simulink model "zynqRadioHWSWLTEDetectorAD9361AD9364SL"  (R2016a)
settings: Solver=FixedStepDiscrete  SolverMode=SingleTasking  StartTime=0.0  StopTime=inf  RelTol=1e-3
InitFcn:
  | % Load LTE detector initialization parameters
  | simParams = hdlcoder_lteofdm_modDetectref_init;
  | simParams = hdlcoder_lteofdm_modDetecthdl_init(simParams);
  | 
  | % Modify PSS detection threshold gain for modified
  | % front-end filter
  | simParams.thresholdGain = 16;
  | 
  | % Load LTE TX waveforms
  | load('zynqRadioLTETransmitData');
libraries: simulink x26, hdlsllib x18, dspsigops x3, dspxfrm3 x1, dspmlti4 x1, dspmathops x1, dspsrcs4 x1
(part 1 of 2)
CloseFcn:
  | clear simParams;
settings Model: DataTypeOverride=Off  SimulationMode=accelerator  Creator=The MathWorks, Inc.  LastModifiedBy=The MathWorks, Inc.
settings DataIOCC: LimitDataPoints=on  SaveFormat=Array  SaveOutput=off  VisualizeSimOutput=off  SaveTime=off
settings OptimizationCC: BlockReduction=off  BooleanDataType=off  ConditionallyExecuteInputs=off  DefaultParameterBehavior=Inlined  EfficientMapNaN2IntZero=off
settings DebuggingCC: AlgebraicLoopMsg=error  SaveWithParameterizedLinksMsg=none  UnderspecifiedInitializationDetection=Classic  MergeDetectMultiDrivingBlocksExec=none  SignalResolutionControl=TryResolveAllWithWarning  SingleTaskRateTransMsg=error  ParameterPrecisionLossMsg=none  AllowSymbolicDim=off  StrictBusMsg=ErrorOnBusTreatedAsVector
settings HardwareCC: ProdBitPerPointer=32  ProdLargestAtomicFloat=None  ProdIntDivRoundTo=Undefined  ProdEndianess=Unspecified  ProdWordSize=32  ProdHWDeviceType=ASIC/FPGA->ASIC/FPGA  TargetBitPerPointer=64  TargetLongLongMode=on  TargetIntDivRoundTo=Zero  TargetEndianess=LittleEndian  TargetWordSize=64  TargetHWDeviceType=MATLAB Host  ProdEqTarget=off
settings ModelReferenceCC: PropagateSignalLabelsOutOfModel=off
settings CodeAppCC: MaxIdLength=128
settings GRTTargetCC: GeneratePreprocessorConditionals=Use local settings  CombineOutputUpdateFcns=off  GRTInterface=on
settings ConfigComp: CovSFcnEnable=off

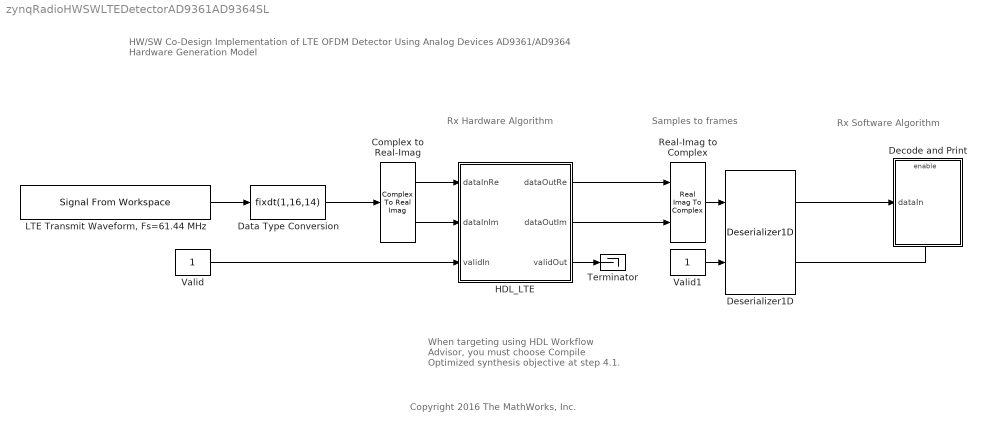
== system zynqRadioHWSWLTEDetectorAD9361AD9364SL ==
  note: When targeting using HDL Workflow Advisor, you must choose Compile Optimized synthesis objective at step 4.1.
  note: HW/SW Co-Design Implementation of LTE OFDM Detector Using Analog Devices AD9361/AD9364
      | Hardware Generation Model
  note: Copyright 2016 The MathWorks, Inc.
  note: Rx Software Algorithm
  note: Rx Hardware Algorithm
  note: Samples to frames
  Complex to Real-Imag : ComplexToRealImag
  Data Type Conversion : DataTypeConversion  OutDataTypeStr=fixdt(1,16,14)
  Decode and Print : Subsystem
  Deserializer1D : hdlsllib/HDL Operations/Deserializer1D  Ratio=5000  IdleCycles=0  InitialCondition=0  startIn=off  validIn=on  validOut=on  inputDataDimensions=1  inputSampleTime=-1  inputSignalType=auto
  HDL_LTE : Subsystem  TreatAsAtomicUnit=on
  "LTE Transmit Waveform, Fs=61.44 MHz" : dspsrcs4/Signal From Workspace  X=zynqRadioLTETransmitData_CellID_16  Ts=1/61.44e6  nsamps=1  OutputAfterFinalValue=Cyclic repetition  ignoreOrWarnInputAndFrameLengths=off  OutputFrames=off
  Real-Imag to Complex : RealImagToComplex
  Terminator : Terminator
  Valid : Constant  VectorParams1D=off  OutDataTypeStr=boolean  SampleTime=1/61.44e6
  Valid1 : Constant  VectorParams1D=off  OutDataTypeStr=boolean  SampleTime=1/61.44e6
  wires:
  "LTE Transmit Waveform, Fs=61.44 MHz"/1 -> Data Type Conversion/1
  Complex to Real-Imag/1 -> HDL_LTE/1(dataInRe)
  Complex to Real-Imag/2 -> HDL_LTE/2(dataInIm)
  HDL_LTE/1(dataOutRe) -> Real-Imag to Complex/1
  HDL_LTE/2(dataOutIm) -> Real-Imag to Complex/2
  Real-Imag to Complex/1 -> Deserializer1D/1
  Deserializer1D/1 -> Decode and Print/1(dataIn)
  Deserializer1D/2 -> Decode and Print/Enable
  Data Type Conversion/1 -> Complex to Real-Imag/1
  Valid/1 -> HDL_LTE/3(validIn)
  Valid1/1 -> Deserializer1D/2
  HDL_LTE/3(validOut) -> Terminator/1

== system zynqRadioHWSWLTEDetectorAD9361AD9364SL/Decode and Print ==
  dataIn : Inport
  Enable : EnablePort
  PrintCellID : MATLAB Function  TreatAsAtomicUnit=on
  wires:
  dataIn/1 -> PrintCellID/1(u)

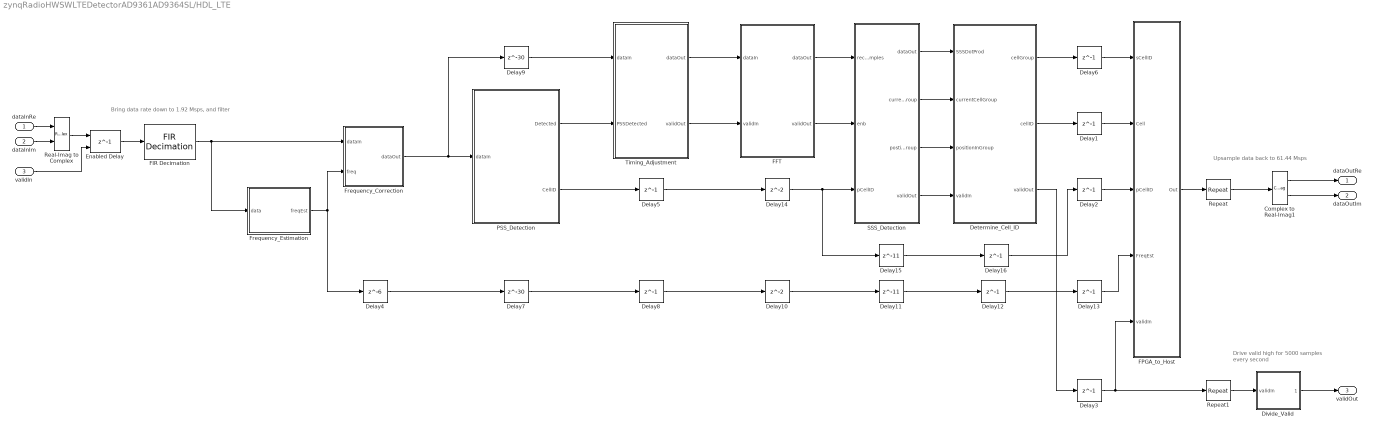
== system zynqRadioHWSWLTEDetectorAD9361AD9364SL/HDL_LTE ==
  note: Drive valid high for 5000 samples
      | every second
  note: Upsample data back to 61.44 Msps
  note: Bring data rate down to 1.92 Msps, and filter
  dataInRe : Inport
  dataInIm : Inport  Port=2
  validIn : Inport  Port=3
  Complex to Real-Imag1 : ComplexToRealImag
  Delay{1..3,5..6,8,12..13,16} (9 alike) : Delay  DelayLength=1  InitialCondition=0  UseCircularBuffer=on
  Delay10 : Delay  InitialCondition=0  UseCircularBuffer=on
  Delay11 : Delay  DelayLength=11  InitialCondition=0  UseCircularBuffer=on
  Delay14 : Delay  InitialCondition=0  UseCircularBuffer=on
  Delay15 : Delay  DelayLength=11  InitialCondition=0  UseCircularBuffer=on
  Delay4 : Delay  DelayLength=6  InitialCondition=0  UseCircularBuffer=on
  Delay7 : Delay  DelayLength=30  InitialCondition=0  InputProcessing=Columns as channels (frame based)
  Delay9 : Delay  DelayLength=30  InitialCondition=0  InputProcessing=Columns as channels (frame based)
  Determine_Cell_ID : Subsystem
  Divide_Valid : Subsystem  mask{cnt=61.44e6, frameSize=5000}
      mask prompts: cnt "Count Value"; frameSize "Frame Size"
  Enabled Delay : Delay  DelayLength=1  ShowEnablePort=on
      settings: InputPortMap=u0,e6
  FFT : Subsystem
  FIR Decimation : dspmlti4/FIR Decimation  FilterSource=Dialog parameters  h="[-0.00658036135584628\t0.0196845728924509\t0.0188740770712237\t0.0238501032851229\t0.0307518159057901\t0.0383679693229666\t0.0461438771533022\t0.0536253945544419\t0.0604305519429808\t0.0661752266061415\t0.0705384318505213\t0.0732639414365212\t0.0741823592553149\t0.0732639414365212\t0.0705384318505213\t0.0661752266061415\t0.0604305519429808\t0.0536253945544419\t0.0461438771533022\t0.0383679693229666\t0.0307518159057901\t0.0238501032851229\t0.0188740770712237\t0.0196845728924509\t-0.00658036135584628]"  D=32  filtStruct=Direct form transposed  FilterObject=FDECIM  framing=Enforce single-rate processing  inputOffset=0  outputBufInitCond=0  roundingMode=Floor  overflowMode=off  firstCoeffDataTypeStr=Inherit: Same word length as input  firstCoeffMin=[]  firstCoeffMax=[]  firstCoeffLastDataTypeStr=Inherit: Same word length as input  outputMin=[]  outputMax=[]
  FPGA_to_Host : Subsystem
  Frequency_Correction : Subsystem
  Frequency_Estimation : Subsystem
  PSS_Detection : Subsystem
  Real-Imag to Complex : RealImagToComplex
  Repeat : dspsigops/Repeat  N=32  RateOptions=Allow multirate processing  ic=0  mode=Unused parameter value
  Repeat1 : dspsigops/Repeat  N=32  RateOptions=Allow multirate processing  ic=0  mode=Unused parameter value
  SSS_Detection : Subsystem
  Timing_Adjustment : Subsystem
  dataOutRe : Outport
  dataOutIm : Outport  Port=2
  validOut : Outport  Port=3  PortDimensions=1
  wires:
  Delay6/1 -> FPGA_to_Host/1(sCellID)
  FPGA_to_Host/1(Out) -> Repeat/1
  Delay1/1 -> FPGA_to_Host/2(Cell)
  Timing_Adjustment/2(validOut) -> FFT/2(validIn)
  FFT/2(validOut) -> SSS_Detection/2(enb)
  Delay9/1 -> Timing_Adjustment/1(dataIn)
  FFT/1(dataOut) -> SSS_Detection/1(receiveSamples)
  Timing_Adjustment/1(dataOut) -> FFT/1(dataIn)
  SSS_Detection/1(dataOut) -> Determine_Cell_ID/1(SSSDotProd)
  SSS_Detection/2(currentCellGroup) -> Determine_Cell_ID/2(currentCellGroup)
  SSS_Detection/3(postionInGroup) -> Determine_Cell_ID/3(positionInGroup)
  PSS_Detection/2(CellID) -> Delay5/1
  PSS_Detection/1(Detected) -> Timing_Adjustment/2(PSSDetected)
  Frequency_Correction/1(dataOut) -> Delay9/1, PSS_Detection/1(dataIn)
  Frequency_Estimation/1(freqEst) -> Frequency_Correction/2(freq), Delay4/1
  Determine_Cell_ID/1(cellGroup) -> Delay6/1
  Determine_Cell_ID/2(cellID) -> Delay1/1
  Delay2/1 -> FPGA_to_Host/3(pCellID)
  Enabled Delay/1 -> FIR Decimation/1
  Real-Imag to Complex/1 -> Enabled Delay/1
  dataInRe/1 -> Real-Imag to Complex/1
  dataInIm/1 -> Real-Imag to Complex/2
  validIn/1 -> Enabled Delay/2
  Repeat/1 -> Complex to Real-Imag1/1
  Complex to Real-Imag1/1 -> dataOutRe/1
  Complex to Real-Imag1/2 -> dataOutIm/1
  SSS_Detection/4(validOut) -> Determine_Cell_ID/4(validIn)
  Determine_Cell_ID/3(validOut) -> Delay3/1
  Delay3/1 -> Repeat1/1, FPGA_to_Host/5(validIn)
  Delay4/1 -> Delay7/1
  Delay7/1 -> Delay8/1
  Delay8/1 -> Delay10/1
  Delay10/1 -> Delay11/1
  Delay11/1 -> Delay12/1
  Delay12/1 -> Delay13/1
  Delay14/1 -> SSS_Detection/3(pCellID), Delay15/1
  Delay15/1 -> Delay16/1
  Delay16/1 -> Delay2/1
  Delay5/1 -> Delay14/1
  Delay13/1 -> FPGA_to_Host/4(FreqEst)
  Divide_Valid/1(validOut) -> validOut/1
  Repeat1/1 -> Divide_Valid/1(validIn)
  FIR Decimation/1 -> Frequency_Estimation/1(data), Frequency_Correction/1(dataIn)

== system zynqRadioHWSWLTEDetectorAD9361AD9364SL/HDL_LTE/Determine_Cell_ID ==
  note: N_ID(2)
  note: Calculate detected Cell ID
      | (CellID = 3*N_ID(1) + N_ID(2))
  note: N_ID(1)
  note: If incoming SSS correlation output is greater than that stored in register,
      | store new maximum value, and cell group number, in registers
  note: Store maximum value in register
  note: Store corresponding cell group in register
  SSSDotProd : Inport
  currentCellGroup : Inport  Port=2
  positionInGroup : Inport  Port=3
  validIn : Inport  Port=4
  Add2 : Sum  OutDataTypeStr=Inherit: Same as first input
  Delay3 : Delay  DelayLength=1  InitialCondition=0  UseCircularBuffer=on
  Gain1 : Gain  Gain=3  OutDataTypeStr=fixdt(0,9,0)
  Relational Operator4 : RelationalOperator  Operator=>  OutDataTypeStr=boolean
  Unit Delay Enabled1 : simulink/Additional Math & Discrete/Additional Discrete/Unit Delay Enabled  vinit=0  tsamp=-1
  Unit Delay Enabled3 : simulink/Additional Math & Discrete/Additional Discrete/Unit Delay Enabled  vinit=0  tsamp=-1
  cellGroup : Outport
  cellID : Outport  Port=2
  validOut : Outport  Port=3
  wires:
  Add2/1 -> cellID/1
  SSSDotProd/1 -> Unit Delay Enabled3/1, Relational Operator4/1
  positionInGroup/1 -> Add2/2
  Unit Delay Enabled1/1 -> Gain1/1, cellGroup/1
  currentCellGroup/1 -> Unit Delay Enabled1/1
  Relational Operator4/1 -> Unit Delay Enabled3/2, Unit Delay Enabled1/2
  Gain1/1 -> Add2/1
  Unit Delay Enabled3/1 -> Relational Operator4/2
  validIn/1 -> Delay3/1
  Delay3/1 -> validOut/1

== system zynqRadioHWSWLTEDetectorAD9361AD9364SL/HDL_LTE/Divide_Valid ==
  validIn : Inport
  Compare To Constant : simulink/Logic and Bit Operations/Compare To Constant  relop=>  const=cnt-frameSize-1  OutDataTypeStr=boolean
  HDL Counter : hdlsllib/HDL Operations/HDL Counter  CountType=Count limited  CountInit=0  CountStep=1  CountMax=cnt-1  CountFromType=Initial value  CountFrom=0  CountResetPort=off  CountLoadPort=off  CountEnbPort=on  CountDirPort=off  CountDataType=Unsigned  CountWordLen=ceil(log2(cnt))  CountFracLen=0  CountSampTime=1
  validOut : Outport
  wires:
  Compare To Constant/1 -> validOut/1
  HDL Counter/1 -> Compare To Constant/1
  validIn/1 -> HDL Counter/1

== system zynqRadioHWSWLTEDetectorAD9361AD9364SL/HDL_LTE/FFT ==
  note: Set input of FFT to input wordlength + FFT growth to allow
      | the output of the FFT to scale. Maximum bit growth is equal
      | to log2(nFFT).
  dataIn : Inport
  validIn : Inport  Port=2
  Data Type Conversion : DataTypeConversion  OutDataTypeStr=fixdt(1,18,10)  RndMeth=Round
  Delay{1..2,4..5} (4 alike) : Delay  DelayLength=1  InitialCondition=0  InputProcessing=Columns as channels (frame based)
  FFT HDL Optimized : dspxfrm3/FFT HDL Optimized  Architecture=Streaming Radix 2 (this choice will be removed -see release notes).  ComplexMultiplication=Use 3 multipliers and 5 adders  BitReversedOutput=off  Normalize=off  FFTLength=128  RoundingMethod=Floor  ResetInputPort=off  StartOutputPort=off  EndOutputPort=off  SimulateUsing=Code generation
  Signal Specification : SignalSpecification  Dimensions=1
  Signal Specification1 : SignalSpecification  Dimensions=1
  dataOut : Outport
  validOut : Outport  Port=2
  wires:
  Signal Specification1/1 -> FFT HDL Optimized/2
  Signal Specification/1 -> FFT HDL Optimized/1
  FFT HDL Optimized/2 -> Delay5/1
  FFT HDL Optimized/1 -> Delay4/1
  Delay4/1 -> Data Type Conversion/1
  Delay2/1 -> Signal Specification1/1
  dataIn/1 -> Delay1/1
  validIn/1 -> Delay2/1
  Delay1/1 -> Signal Specification/1
  Data Type Conversion/1 -> dataOut/1
  Delay5/1 -> validOut/1

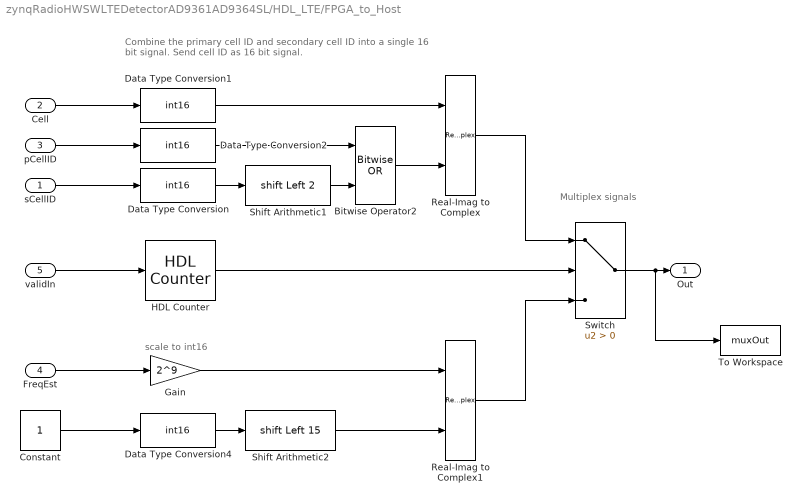
== system zynqRadioHWSWLTEDetectorAD9361AD9364SL/HDL_LTE/FPGA_to_Host ==
  note: Multiplex signals
  note: scale to int16
  note: Combine the primary cell ID and secondary cell ID into a single 16 bit signal. Send cell ID as 16 bit signal.
  sCellID : Inport
  Cell : Inport  Port=2
  pCellID : Inport  Port=3
  FreqEst : Inport  Port=4
  validIn : Inport  Port=5
  Bitwise Operator2 : simulink/Logic and Bit Operations/Bitwise Operator  logicop=OR  UseBitMask=off  NumInputPorts=2  BitMask=bin2dec('11011001')  BitMaskRealWorld=Stored Integer
  Constant : Constant  VectorParams1D=off  OutDataTypeStr=boolean  SampleTime=-1
  Data Type Conversion{,1..2,4} (4 alike) : DataTypeConversion  OutDataTypeStr=int16
  Gain : Gain  Gain=2^9  OutDataTypeStr=int16
  HDL Counter : hdlsllib/HDL Operations/HDL Counter  CountType=Count limited  CountInit=0  CountStep=1  CountMax=1  CountFromType=Initial value  CountFrom=0  CountResetPort=off  CountLoadPort=off  CountEnbPort=on  CountDirPort=off  CountDataType=Unsigned  CountWordLen=1  CountFracLen=0  CountSampTime=1
  Real-Imag to Complex : RealImagToComplex
  Real-Imag to Complex1 : RealImagToComplex
  Shift Arithmetic1 : ArithShift  BitShiftNumber=2  BitShiftDirection=Left
  Shift Arithmetic2 : ArithShift  BitShiftNumber=15  BitShiftDirection=Left
  Switch : Switch  Criteria=u2 > Threshold
  To Workspace : ToWorkspace  VariableName=muxOut  SampleTime=-1
      settings: Save2DSignal=2-D array (concatenate along first dimension)
  Out : Outport
  wires:
  Data Type Conversion2/1 -> Bitwise Operator2/1
  Data Type Conversion/1 -> Shift Arithmetic1/1
  Bitwise Operator2/1 -> Real-Imag to Complex/2
  Shift Arithmetic1/1 -> Bitwise Operator2/2
  Data Type Conversion1/1 -> Real-Imag to Complex/1
  Cell/1 -> Data Type Conversion1/1
  sCellID/1 -> Data Type Conversion/1
  pCellID/1 -> Data Type Conversion2/1
  Switch/1 -> To Workspace/1, Out/1
  FreqEst/1 -> Gain/1
  validIn/1 -> HDL Counter/1
  HDL Counter/1 -> Switch/2
  Real-Imag to Complex/1 -> Switch/1
  Gain/1 -> Real-Imag to Complex1/1
  Shift Arithmetic2/1 -> Real-Imag to Complex1/2
  Constant/1 -> Data Type Conversion4/1
  Data Type Conversion4/1 -> Shift Arithmetic2/1
  Real-Imag to Complex1/1 -> Switch/3

== system zynqRadioHWSWLTEDetectorAD9361AD9364SL/HDL_LTE/Frequency_Correction ==
  note: This subsystem corrects the frequency offset using an Numerically Controller Oscillator (NCO) and a conjugate multiplication.
  dataIn : Inport
  freq : Inport  Port=2
  Data Type Conversion : DataTypeConversion  OutDataTypeStr=fixdt(1,16,15)  RndMeth=Nearest
  Delay{1..6} (6 alike) : Delay  DelayLength=1  InitialCondition=0  UseCircularBuffer=on
  Gain : Gain  Gain=2^9  OutDataTypeStr=int16
  NCO HDL Optimized : dspsigops/NCO HDL Optimized  PhaseIncrementSource=Input port  PhaseIncrement=100  PhaseOffsetSource=Property  PhaseOffset=0  DitherSource=Property  NumDitherBits=4  PhaseQuantization=on  NumQuantizerAccumulatorBits=12  LUTCompress=on  ResetAction=off  ValidInputPort=off  Waveform=Complex exponential  PhasePort=off  AccumulatorWL=16  OutputDataType=Binary point scaling  OutputWL=16  OutputFL=14  SimulateUsing=Code generation
  Product1 : Product
  Signal Spec : SignalSpecification  Dimensions=1
  Unit Delay Enabled : simulink/Additional Math & Discrete/Additional Discrete/Unit Delay Enabled  vinit=0.0  tsamp=-1
  complexConjugate : Math  Operator=conj  SaturateOnIntegerOverflow=on
  dataOut : Outport
  wires:
  complexConjugate/1 -> Delay3/1
  NCO HDL Optimized/2 -> Unit Delay Enabled/2
  dataIn/1 -> Delay2/1
  Product1/1 -> Delay4/1
  NCO HDL Optimized/1 -> Unit Delay Enabled/1
  Unit Delay Enabled/1 -> complexConjugate/1
  Data Type Conversion/1 -> Delay1/1
  Delay2/1 -> Product1/1
  Delay1/1 -> dataOut/1
  Delay4/1 -> Data Type Conversion/1
  Delay3/1 -> Product1/2
  Gain/1 -> Delay5/1
  freq/1 -> Delay6/1
  Delay6/1 -> Gain/1
  Signal Spec/1 -> NCO HDL Optimized/1
  Delay5/1 -> Signal Spec/1

== system zynqRadioHWSWLTEDetectorAD9361AD9364SL/HDL_LTE/Frequency_Estimation ==
  data : Inport
  Angle_Filter : Subsystem
  Angle_at_Maximum : Subsystem
  Cyclic_Prefix_Correlator : Subsystem
  Rect_to_Polar : Subsystem
  freqEst : Outport
  wires:
  data/1 -> Cyclic_Prefix_Correlator/1(dataIn)
  Rect_to_Polar/3(validOut) -> Angle_at_Maximum/3(validIn)
  Angle_at_Maximum/1(angleOut) -> Angle_Filter/1(angleIn)
  Rect_to_Polar/2(angleOut) -> Angle_at_Maximum/2(angleIn)
  Rect_to_Polar/1(magOut) -> Angle_at_Maximum/1(magIn)
  Cyclic_Prefix_Correlator/1(corrOut) -> Rect_to_Polar/1(dataIn)
  Angle_Filter/1(angleOut) -> freqEst/1
  Angle_at_Maximum/2(validOut) -> Angle_Filter/2(en)

== system zynqRadioHWSWLTEDetectorAD9361AD9364SL/HDL_LTE/PSS_Detection ==
  dataIn : Inport
  Cross_Correlation : Subsystem
  Determine_Primary_Cell_ID : Subsystem
  Peak_Detection : Subsystem
  Detected : Outport
  CellID : Outport  Port=2
  wires:
  Determine_Primary_Cell_ID/1(Cell_ID) -> CellID/1
  Determine_Primary_Cell_ID/2(PSSDetected) -> Detected/1
  Cross_Correlation/1(PSS0) -> Peak_Detection/1(PSS0)
  Cross_Correlation/2(PSS1) -> Peak_Detection/2(PSS1)
  Cross_Correlation/3(PSS2) -> Peak_Detection/3(PSS2)
  Cross_Correlation/4(Threshold) -> Peak_Detection/4(thresholdIn)
  Peak_Detection/2(PSS0Strength) -> Determine_Primary_Cell_ID/2(PSS0Strength)
  Peak_Detection/4(PSS1Strength) -> Determine_Primary_Cell_ID/4(PSS1Strength)
  Peak_Detection/5(PSS2Detected) -> Determine_Primary_Cell_ID/5(PSS2Detected)
  Peak_Detection/6(PSS2Strength) -> Determine_Primary_Cell_ID/6(PSS2Strength)
  Peak_Detection/1(PSS0Detected) -> Determine_Primary_Cell_ID/1(PSS0Detected)
  Peak_Detection/3(PSS1Detected) -> Determine_Primary_Cell_ID/3(PSS1Detected)
  dataIn/1 -> Cross_Correlation/1(dataIn)

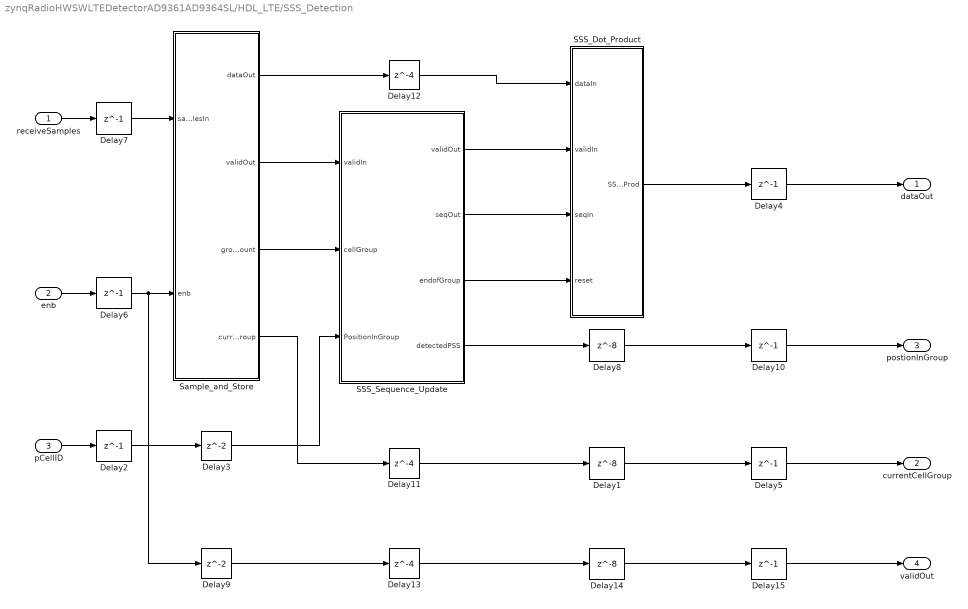
== system zynqRadioHWSWLTEDetectorAD9361AD9364SL/HDL_LTE/SSS_Detection ==
  receiveSamples : Inport
  enb : Inport  Port=2
  pCellID : Inport  Port=3
  Delay1 : Delay  DelayLength=8  InitialCondition=0  UseCircularBuffer=on
  Delay{2,4..7,10,15} (7 alike) : Delay  DelayLength=1  InitialCondition=0  UseCircularBuffer=on
  Delay11 : Delay  DelayLength=4  InitialCondition=0
  Delay12 : Delay  DelayLength=4  InitialCondition=0
  Delay13 : Delay  DelayLength=4  InitialCondition=0
  Delay14 : Delay  DelayLength=8  InitialCondition=0  UseCircularBuffer=on
  Delay3 : Delay  InitialCondition=0
  Delay8 : Delay  DelayLength=8  InitialCondition=0  UseCircularBuffer=on
  Delay9 : Delay  InitialCondition=0
  SSS_Dot_Product : Subsystem
  SSS_Sequence_Update : Subsystem
  Sample_and_Store : Subsystem
  dataOut : Outport
  currentCellGroup : Outport  Port=2
  postionInGroup : Outport  Port=3
  validOut : Outport  Port=4
  wires:
  SSS_Dot_Product/1(SSSDotProd) -> Delay4/1
  Delay3/1 -> SSS_Sequence_Update/3(PositionInGroup)
  Sample_and_Store/3(groupCount) -> SSS_Sequence_Update/2(cellGroup)
  Delay2/1 -> Delay3/1
  enb/1 -> Delay6/1
  receiveSamples/1 -> Delay7/1
  pCellID/1 -> Delay2/1
  Sample_and_Store/2(validOut) -> SSS_Sequence_Update/1(validIn)
  Delay7/1 -> Sample_and_Store/1(samplesIn)
  Delay6/1 -> Delay9/1, Sample_and_Store/2(enb)
  Sample_and_Store/1(dataOut) -> Delay12/1
  SSS_Sequence_Update/1(validOut) -> SSS_Dot_Product/2(validIn)
  SSS_Sequence_Update/2(seqOut) -> SSS_Dot_Product/3(seqIn)
  SSS_Sequence_Update/3(endofGroup) -> SSS_Dot_Product/4(reset)
  SSS_Sequence_Update/4(detectedPSS) -> Delay8/1
  Delay8/1 -> Delay10/1
  Delay1/1 -> Delay5/1
  Delay10/1 -> postionInGroup/1
  Delay5/1 -> currentCellGroup/1
  Delay4/1 -> dataOut/1
  Sample_and_Store/4(currentCellGroup) -> Delay11/1
  Delay11/1 -> Delay1/1
  Delay12/1 -> SSS_Dot_Product/1(dataIn)
  Delay9/1 -> Delay13/1
  Delay13/1 -> Delay14/1
  Delay14/1 -> Delay15/1
  Delay15/1 -> validOut/1

== system zynqRadioHWSWLTEDetectorAD9361AD9364SL/HDL_LTE/Timing_Adjustment ==
  note: Detect PSS detection strobe, and create
      | valid high signal.
  note: Delay signal so that once the PSS
      | has been detected, the resource block
      | containing the SSS signal (the previous
      | block) is aligned here.
  note: Only output samples once
      | the detected strobe has
      | been received.
  note: PSS detect strobe is high at the end of the PSS
      | sequence, so delay must be for the full 128 samples
      | of the PSS, and the full 128 samples of the SSS, plus
      | a single short CP length of 9 samples for 128-point
      | FFT.
  dataIn : Inport
  PSSDetected : Inport  Port=2
  Constant : Constant  Value=complex(0)  OutDataTypeStr=fixdt(1,16,15)  SampleTime=simParams.TsRx
  Constant1 : Constant  OutDataTypeStr=boolean  SampleTime=simParams.TsRx
  Delay1 : Delay  DelayLength=265  InitialCondition=0  InputProcessing=Columns as channels (frame based)
  Delay{2..5} (4 alike) : Delay  DelayLength=1  InitialCondition=0  UseCircularBuffer=on
  Switch : Switch  Criteria=u2 > Threshold
  Unit Delay Enabled1 : simulink/Additional Math & Discrete/Additional Discrete/Unit Delay Enabled  vinit=0.0  tsamp=-1
  dataOut : Outport
  validOut : Outport  Port=2
  wires:
  Delay5/1 -> validOut/1
  Delay4/1 -> dataOut/1
  Delay3/1 -> Delay1/1
  Delay2/1 -> Unit Delay Enabled1/2
  Constant/1 -> Switch/3
  Delay1/1 -> Switch/1
  dataIn/1 -> Delay3/1
  Switch/1 -> Delay4/1
  PSSDetected/1 -> Delay2/1
  Unit Delay Enabled1/1 -> Switch/2, Delay5/1
  Constant1/1 -> Unit Delay Enabled1/1

== system zynqRadioHWSWLTEDetectorAD9361AD9364SL/HDL_LTE/Frequency_Estimation/Angle_Filter ==
  note: This subsystem implements a 1-pole IIR filter to perform further averaging of the correlation angle results. The filter's gain is normalized to 0dB and an efficient implementation which requires only 1 multiplier is used.
  angleIn : Inport
  en : Inport  Port=2
  Add : Sum  Inputs=|-+
  Add1 : Sum  Inputs=|-+
  Delay1 : Delay  DelayLength=1  InitialCondition=0  UseCircularBuffer=on
  Delay2 : Delay  DelayLength=1  InitialCondition=0  UseCircularBuffer=on
  Delay3 : Delay  DelayLength=1  InitialCondition=0  UseCircularBuffer=on
  Gain : Gain  Gain=2^-2  OutDataTypeStr=Inherit: Same as input
  Unit Delay Enabled : simulink/Additional Math & Discrete/Additional Discrete/Unit Delay Enabled  vinit=0.0  tsamp=-1
  angleOut : Outport
  wires:
  angleIn/1 -> Delay2/1
  Add/1 -> Gain/1
  Gain/1 -> Add1/1
  Unit Delay Enabled/1 -> Add/2, Add1/2, Delay1/1
  Add1/1 -> Unit Delay Enabled/1
  en/1 -> Delay3/1
  Delay1/1 -> angleOut/1
  Delay2/1 -> Add/1
  Delay3/1 -> Unit Delay Enabled/2

== system zynqRadioHWSWLTEDetectorAD9361AD9364SL/HDL_LTE/Frequency_Estimation/Angle_at_Maximum ==
  note: This subsystem records the maximum CP correlation level, and the corresponding phase angle of the result, across windows of time equivalent to 1 slot (960 samples). A counter is used to reset the running max and record the final phase value, which is then passed to the output and qualified by the validOut signal.
  note: Store current mag & angle if mag is greater than previous max mag.
  note: This register stores the current running max magnitude in the current time window
  magIn : Inport
  angleIn : Inport  Port=2
  validIn : Inport  Port=3
  Compare To Constant : simulink/Logic and Bit Operations/Compare To Constant  relop===  const=0  OutDataTypeStr=boolean
  Delay{1..3,5} (4 alike) : Delay  DelayLength=1  InitialCondition=0  UseCircularBuffer=on
  HDL Counter : hdlsllib/HDL Operations/HDL Counter  CountType=Count limited  CountInit=0  CountStep=1  CountMax=959  CountFromType=Initial value  CountFrom=0  CountResetPort=off  CountLoadPort=off  CountEnbPort=on  CountDirPort=off  CountDataType=Unsigned  CountWordLen=10  CountFracLen=0  CountSampTime=1
  Logical Operator : Logic  Operator=OR  IconShape=distinctive  AllPortsSameDT=off  OutDataTypeStr=boolean
  Relational Operator : RelationalOperator  Operator=>  OutDataTypeStr=boolean
  Unit Delay Enabled : simulink/Additional Math & Discrete/Additional Discrete/Unit Delay Enabled  vinit=0.0  tsamp=-1
  Unit Delay Enabled1 : simulink/Additional Math & Discrete/Additional Discrete/Unit Delay Enabled  vinit=0.0  tsamp=-1
  Unit Delay Enabled2 : simulink/Additional Math & Discrete/Additional Discrete/Unit Delay Enabled  vinit=0.0  tsamp=-1
  angleOut : Outport
  validOut : Outport  Port=2
  wires:
  magIn/1 -> Delay5/1
  angleIn/1 -> Delay1/1
  HDL Counter/1 -> Compare To Constant/1
  Compare To Constant/1 -> Unit Delay Enabled2/2, Logical Operator/2, Delay3/1
  Unit Delay Enabled1/1 -> Unit Delay Enabled2/1
  validIn/1 -> Delay2/1
  Delay5/1 -> Relational Operator/1, Unit Delay Enabled/1
  Delay2/1 -> HDL Counter/1
  Unit Delay Enabled2/1 -> angleOut/1
  Delay3/1 -> validOut/1
  Unit Delay Enabled/1 -> Relational Operator/2
  Relational Operator/1 -> Logical Operator/1
  Logical Operator/1 -> Unit Delay Enabled1/2, Unit Delay Enabled/2
  Delay1/1 -> Unit Delay Enabled1/1

== system zynqRadioHWSWLTEDetectorAD9361AD9364SL/HDL_LTE/Frequency_Estimation/Cyclic_Prefix_Correlator ==
  note: Correlate the signal with itself
      | delayed by the FFT length (128 samples).
  note: Integrate across part of the CP length, which is 9 samples. However we use 8 samples here to optimize for HDL implementation.
  note: Finally average across 7 OFDM symbols, i.e. the number in
      | each slot.
  dataIn : Inport
  Delay1 : Delay  DelayLength=1  InitialCondition=0  UseCircularBuffer=on
  Delay2 : Delay  DelayLength=128  InitialCondition=0
  Delay3 : Delay  DelayLength=1  InitialCondition=0  UseCircularBuffer=on
  Delay5 : Delay  DelayLength=1  InitialCondition=0  UseCircularBuffer=on
  Moving_Average : Subsystem
  Product : Product  OutDataTypeStr=fixdt(1,24,23)  RndMeth=Round
  Slot_Average : Subsystem
  complexConj : Math  Operator=conj  SaturateOnIntegerOverflow=on
  corrOut : Outport
  wires:
  Product/1 -> Delay5/1
  Delay3/1 -> Product/2
  Delay2/1 -> complexConj/1
  Slot_Average/1(dataOut) -> corrOut/1
  Moving_Average/1(dataOut) -> Slot_Average/1(dataIn)
  complexConj/1 -> Delay3/1
  Delay5/1 -> Moving_Average/1(dataIn)
  Delay1/1 -> Product/1
  dataIn/1 -> Delay2/1, Delay1/1

== system zynqRadioHWSWLTEDetectorAD9361AD9364SL/HDL_LTE/Frequency_Estimation/Rect_to_Polar ==
  dataIn : Inport
  Complex to Magnitude-Angle HDL Optimized : dspmathops/Complex to Magnitude-Angle HDL Optimized  NumIterationsSource=Auto  NumIterations=16  OutputFormat=Magnitude and angle  AngleFormat=Normalized  ScaleOutput=on  SimulateUsing=Code generation
  Constant : Constant  OutDataTypeStr=boolean  SampleTime=simParams.TsRx
  Delay1 : Delay  InitialCondition=0  UseCircularBuffer=on
  Delay2 : Delay  DelayLength=1  InitialCondition=0  UseCircularBuffer=on
  Delay3 : Delay  DelayLength=1  InitialCondition=0  UseCircularBuffer=on
  Delay4 : Delay  DelayLength=1  InitialCondition=0  UseCircularBuffer=on
  Delay5 : Delay  InitialCondition=0  UseCircularBuffer=on
  Gain : Gain  Gain=0.5  OutDataTypeStr=fixdt(1,27,27)
  Signal Specification1 : SignalSpecification  Dimensions=1
  magOut : Outport
  angleOut : Outport  Port=2
  validOut : Outport  Port=3
  wires:
  Gain/1 -> angleOut/1
  dataIn/1 -> Signal Specification1/1
  Constant/1 -> Delay1/1
  Delay5/1 -> Complex to Magnitude-Angle HDL Optimized/1
  Delay1/1 -> Complex to Magnitude-Angle HDL Optimized/2
  Delay2/1 -> magOut/1
  Delay3/1 -> Gain/1
  Delay4/1 -> validOut/1
  Complex to Magnitude-Angle HDL Optimized/1 -> Delay2/1
  Complex to Magnitude-Angle HDL Optimized/3 -> Delay4/1
  Complex to Magnitude-Angle HDL Optimized/2 -> Delay3/1
  Signal Specification1/1 -> Delay5/1

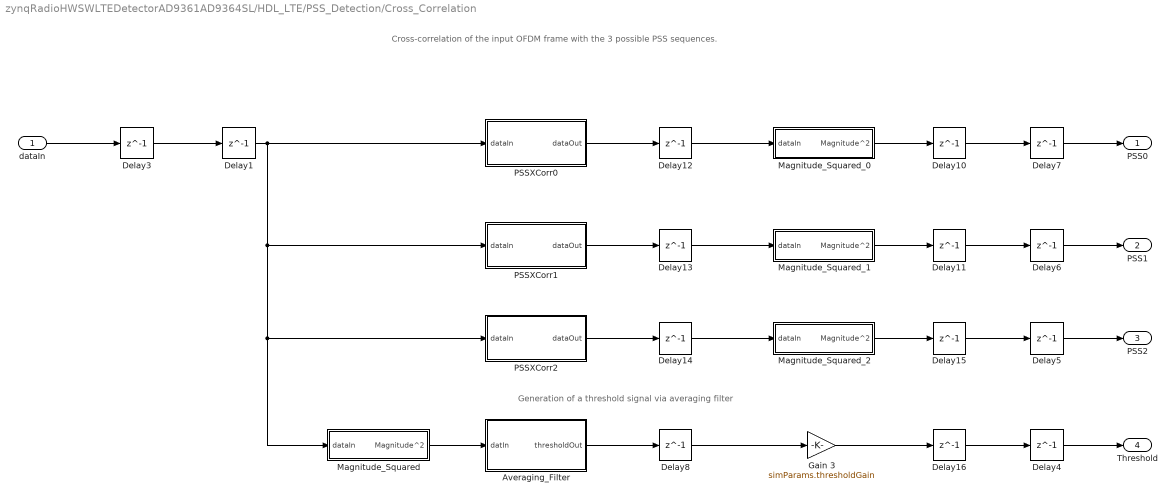
== system zynqRadioHWSWLTEDetectorAD9361AD9364SL/HDL_LTE/PSS_Detection/Cross_Correlation ==
  note: Cross-correlation of the input OFDM frame with the 3 possible PSS sequences.
  note: Generation of a threshold signal via averaging filter
  dataIn : Inport
  Averaging_Filter : Subsystem
  Delay{1,3..8,10..16} (14 alike) : Delay  DelayLength=1  InitialCondition=0
  Gain 3 : Gain  Gain=simParams.thresholdGain  OutDataTypeStr=fixdt(1,32,20)
  Magnitude_Squared : Subsystem
  Magnitude_Squared_0 : Subsystem
  Magnitude_Squared_1 : Subsystem
  Magnitude_Squared_2 : Subsystem
  PSSXCorr0 : Subsystem  mask(ComplexFIRFilter){PSSIdx=0}
      mask prompts: PSSIdx "PSS Sequence (0, 1, 2)"
      mask help: Implements a complex valued FIR filter.
  PSSXCorr1 : Subsystem  mask(ComplexFIRFilter){PSSIdx=1}
      mask prompts: PSSIdx "PSS Sequence (0, 1, 2)"
      mask help: Implements a complex valued FIR filter.
  PSSXCorr2 : Subsystem  mask(ComplexFIRFilter){PSSIdx=2}
      mask prompts: PSSIdx "PSS Sequence (0, 1, 2)"
      mask help: Implements a complex valued FIR filter.
  PSS0 : Outport
  PSS1 : Outport  Port=2
  PSS2 : Outport  Port=3
  Threshold : Outport  Port=4
  wires:
  dataIn/1 -> Delay3/1
  Delay10/1 -> Delay7/1
  Delay11/1 -> Delay6/1
  Delay15/1 -> Delay5/1
  Delay16/1 -> Delay4/1
  Delay4/1 -> Threshold/1
  Delay5/1 -> PSS2/1
  Delay6/1 -> PSS1/1
  Delay7/1 -> PSS0/1
  Delay3/1 -> Delay1/1
  Delay1/1 -> PSSXCorr0/1(dataIn), PSSXCorr1/1(dataIn), PSSXCorr2/1(dataIn), Magnitude_Squared/1(dataIn)
  Delay12/1 -> Magnitude_Squared_0/1(dataIn)
  PSSXCorr0/1(dataOut) -> Delay12/1
  Magnitude_Squared_0/1(Magnitude^2) -> Delay10/1
  Delay13/1 -> Magnitude_Squared_1/1(dataIn)
  PSSXCorr1/1(dataOut) -> Delay13/1
  Magnitude_Squared_1/1(Magnitude^2) -> Delay11/1
  Delay14/1 -> Magnitude_Squared_2/1(dataIn)
  PSSXCorr2/1(dataOut) -> Delay14/1
  Magnitude_Squared_2/1(Magnitude^2) -> Delay15/1
  Magnitude_Squared/1(Magnitude^2) -> Averaging_Filter/1(datIn)
  Averaging_Filter/1(thresholdOut) -> Delay8/1
  Delay8/1 -> Gain 3/1
  Gain 3/1 -> Delay16/1

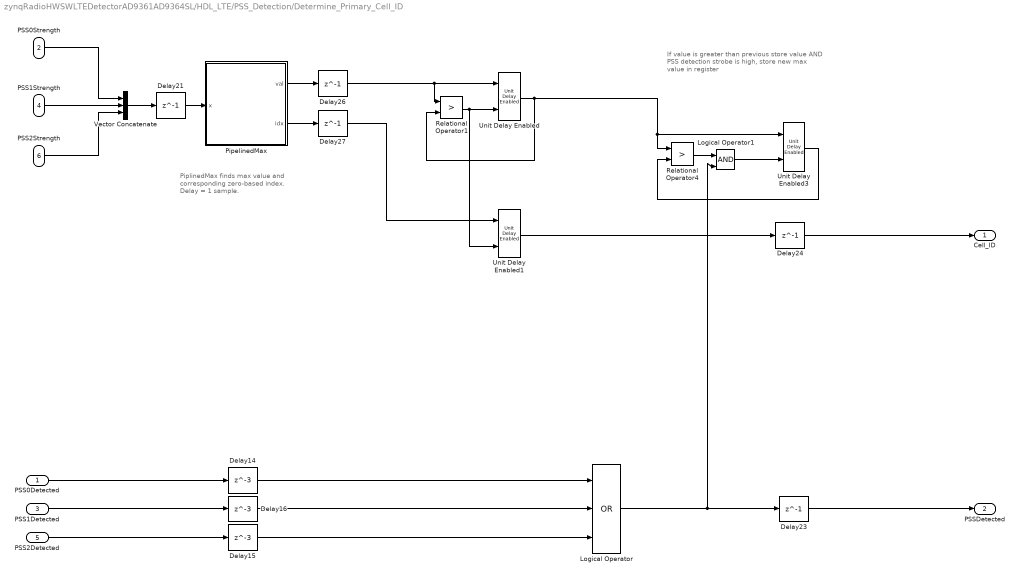
== system zynqRadioHWSWLTEDetectorAD9361AD9364SL/HDL_LTE/PSS_Detection/Determine_Primary_Cell_ID ==
  note: If value is greater than previous store value
      | AND PSS detection strobe is high,
      | store new max value in register
  note: PiplinedMax finds max value and
      | corresponding zero-based index.
      | Delay = 1 sample.
  PSS0Detected : Inport
  PSS0Strength : Inport  Port=2
  PSS1Detected : Inport  Port=3
  PSS1Strength : Inport  Port=4
  PSS2Detected : Inport  Port=5
  PSS2Strength : Inport  Port=6
  Delay14 : Delay  DelayLength=3  InitialCondition=0  InputProcessing=Columns as channels (frame based)
  Delay15 : Delay  DelayLength=3  InitialCondition=0  InputProcessing=Columns as channels (frame based)
  Delay16 : Delay  DelayLength=3  InitialCondition=0  InputProcessing=Columns as channels (frame based)
  Delay{21,23..24,26..27} (5 alike) : Delay  DelayLength=1  InitialCondition=0  InputProcessing=Columns as channels (frame based)
  Logical Operator : Logic  Operator=OR  Inputs=3  IconShape=distinctive  AllPortsSameDT=off  OutDataTypeStr=boolean
  Logical Operator1 : Logic  IconShape=distinctive  AllPortsSameDT=off  OutDataTypeStr=boolean
  PipelinedMax : MATLAB Function  TreatAsAtomicUnit=on
  Relational Operator1 : RelationalOperator  Operator=>  OutDataTypeStr=boolean
  Relational Operator4 : RelationalOperator  Operator=>  OutDataTypeStr=boolean
  Unit Delay Enabled : simulink/Additional Math & Discrete/Additional Discrete/Unit Delay Enabled  vinit=0.0  tsamp=-1
  Unit Delay Enabled1 : simulink/Additional Math & Discrete/Additional Discrete/Unit Delay Enabled  vinit=0.0  tsamp=-1
  Unit Delay Enabled3 : simulink/Additional Math & Discrete/Additional Discrete/Unit Delay Enabled  vinit=0.0  tsamp=-1
  Vector Concatenate : Concatenate  NumInputs=3  Mode=Multidimensional array  ConcatenateDimension=2
  Cell_ID : Outport
  PSSDetected : Outport  Port=2
  wires:
  PSS0Strength/1 -> Vector Concatenate/1
  Relational Operator1/1 -> Unit Delay Enabled1/2, Unit Delay Enabled/2
  PSS2Strength/1 -> Vector Concatenate/3
  Unit Delay Enabled1/1 -> Delay24/1
  PSS2Detected/1 -> Delay15/1
  PSS0Detected/1 -> Delay14/1
  PSS1Detected/1 -> Delay16/1
  Unit Delay Enabled/1 -> Relational Operator1/2, Unit Delay Enabled3/1, Relational Operator4/1
  Unit Delay Enabled3/1 -> Relational Operator4/2
  Logical Operator/1 -> Logical Operator1/2, Delay23/1
  Logical Operator1/1 -> Unit Delay Enabled3/2
  Relational Operator4/1 -> Logical Operator1/1
  PSS1Strength/1 -> Vector Concatenate/2
  Delay23/1 -> PSSDetected/1
  Delay24/1 -> Cell_ID/1
  PipelinedMax/2(idx) -> Delay27/1
  Delay26/1 -> Relational Operator1/1, Unit Delay Enabled/1
  Delay27/1 -> Unit Delay Enabled1/1
  Vector Concatenate/1 -> Delay21/1
  PipelinedMax/1(val) -> Delay26/1
  Delay15/1 -> Logical Operator/3
  Delay16/1 -> Logical Operator/2
  Delay14/1 -> Logical Operator/1
  Delay21/1 -> PipelinedMax/1(x)

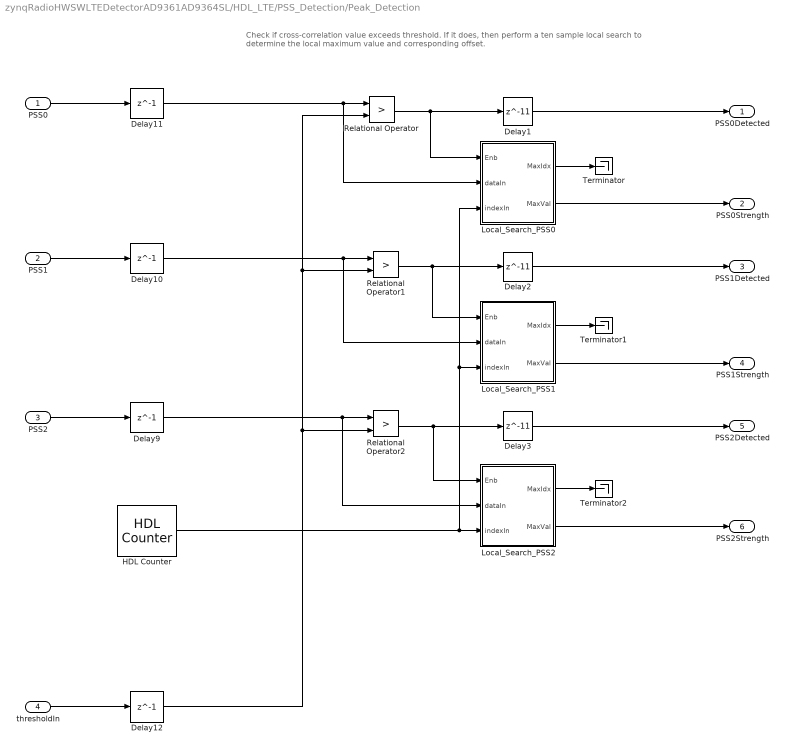
== system zynqRadioHWSWLTEDetectorAD9361AD9364SL/HDL_LTE/PSS_Detection/Peak_Detection ==
  note: Check if cross-correlation value exceeds threshold. If it does, then perform a ten sample local search to determine the local maximum value and corresponding offset.
  PSS0 : Inport
  PSS1 : Inport  Port=2
  PSS2 : Inport  Port=3
  thresholdIn : Inport  Port=4
  Delay1 : Delay  DelayLength=11  InitialCondition=0
  Delay{9..12} (4 alike) : Delay  DelayLength=1  InitialCondition=0  UseCircularBuffer=on
  Delay2 : Delay  DelayLength=11  InitialCondition=0
  Delay3 : Delay  DelayLength=11  InitialCondition=0
  HDL Counter : hdlsllib/HDL Operations/HDL Counter  CountType=Count limited  CountInit=0  CountStep=1  CountMax=19199  CountFromType=Initial value  CountFrom=0  CountResetPort=off  CountLoadPort=off  CountEnbPort=off  CountDirPort=off  CountDataType=Unsigned  CountWordLen=ceil(log2(19199))  CountFracLen=0  CountSampTime=simParams.TsRx
  Local_Search_PSS0 : Subsystem
  Local_Search_PSS1 : Subsystem
  Local_Search_PSS2 : Subsystem
  Relational Operator : RelationalOperator  Operator=>  OutDataTypeStr=boolean
  Relational Operator1 : RelationalOperator  Operator=>  OutDataTypeStr=boolean
  Relational Operator2 : RelationalOperator  Operator=>  OutDataTypeStr=boolean
  Terminator : Terminator
  Terminator1 : Terminator
  Terminator2 : Terminator
  PSS0Detected : Outport
  PSS0Strength : Outport  Port=2
  PSS1Detected : Outport  Port=3
  PSS1Strength : Outport  Port=4
  PSS2Detected : Outport  Port=5
  PSS2Strength : Outport  Port=6
  wires:
  thresholdIn/1 -> Delay12/1
  PSS2/1 -> Delay9/1
  PSS1/1 -> Delay10/1
  Relational Operator/1 -> Delay1/1, Local_Search_PSS0/1(Enb)
  Relational Operator1/1 -> Local_Search_PSS1/1(Enb), Delay2/1
  Relational Operator2/1 -> Local_Search_PSS2/1(Enb), Delay3/1
  PSS0/1 -> Delay11/1
  Local_Search_PSS0/2(MaxVal) -> PSS0Strength/1
  Local_Search_PSS1/2(MaxVal) -> PSS1Strength/1
  Local_Search_PSS2/2(MaxVal) -> PSS2Strength/1
  Delay1/1 -> PSS0Detected/1
  Delay2/1 -> PSS1Detected/1
  Delay3/1 -> PSS2Detected/1
  HDL Counter/1 -> Local_Search_PSS2/3(indexIn), Local_Search_PSS1/3(indexIn), Local_Search_PSS0/3(indexIn)
  Delay9/1 -> Local_Search_PSS2/2(dataIn), Relational Operator2/1
  Delay10/1 -> Local_Search_PSS1/2(dataIn), Relational Operator1/1
  Delay11/1 -> Local_Search_PSS0/2(dataIn), Relational Operator/1
  Delay12/1 -> Relational Operator/2, Relational Operator1/2, Relational Operator2/2
  Local_Search_PSS0/1(MaxIdx) -> Terminator/1
  Local_Search_PSS1/1(MaxIdx) -> Terminator1/1
  Local_Search_PSS2/1(MaxIdx) -> Terminator2/1

== system zynqRadioHWSWLTEDetectorAD9361AD9364SL/HDL_LTE/SSS_Detection/SSS_Dot_Product ==
  note: Accumulate
  note: Reset register after all 63 samples have been processed
  note: Multiply dataIn by seqIn:
      | since seqIn is always either -1 or 1, use a gain of -1 and a switch to invert dataIn when seqIn = -1.
  dataIn : Inport
  validIn : Inport  Port=2
  seqIn : Inport  Port=3
  reset : Inport  Port=4
  Add : Sum  OutDataTypeStr=Inherit: Same as first input
  Compare To Zero1 : simulink/Logic and Bit Operations/Compare To Zero  relop=<  OutDataTypeStr=boolean
  Data Type Conversion : DataTypeConversion  OutDataTypeStr=fixdt(1,24,10)
  Data Type Conversion1 : DataTypeConversion  OutDataTypeStr=fixdt(1,18,4)  RndMeth=Round
  Delay Reset : Subsystem
  Delay1 : Delay  DelayLength=1  InitialCondition=0
  Delay3 : Delay  InitialCondition=0
  Delay5 : Delay  DelayLength=1  InitialCondition=0
  Gain : Gain  Gain=-1  OutDataTypeStr=Inherit: Same as input
  Magnitude Squared 0 : Subsystem
  real1 : Switch  Criteria=u2 ~= 0
  SSSDotProd : Outport  InitialOutput=0
  wires:
  Delay3/1 -> Delay Reset/3(R)
  Delay5/1 -> Delay Reset/2(E)
  Add/1 -> Delay Reset/1(u)
  validIn/1 -> Delay5/1
  Delay1/1 -> Data Type Conversion/1
  Magnitude Squared 0/1(Magnitude^2) -> SSSDotProd/1
  reset/1 -> Delay3/1
  Delay Reset/1(y) -> Add/2, Data Type Conversion1/1
  Data Type Conversion/1 -> Add/1
  real1/1 -> Delay1/1
  dataIn/1 -> Gain/1, real1/3
  Gain/1 -> real1/1
  seqIn/1 -> Compare To Zero1/1
  Compare To Zero1/1 -> real1/2
  Data Type Conversion1/1 -> Magnitude Squared 0/1(dataIn)

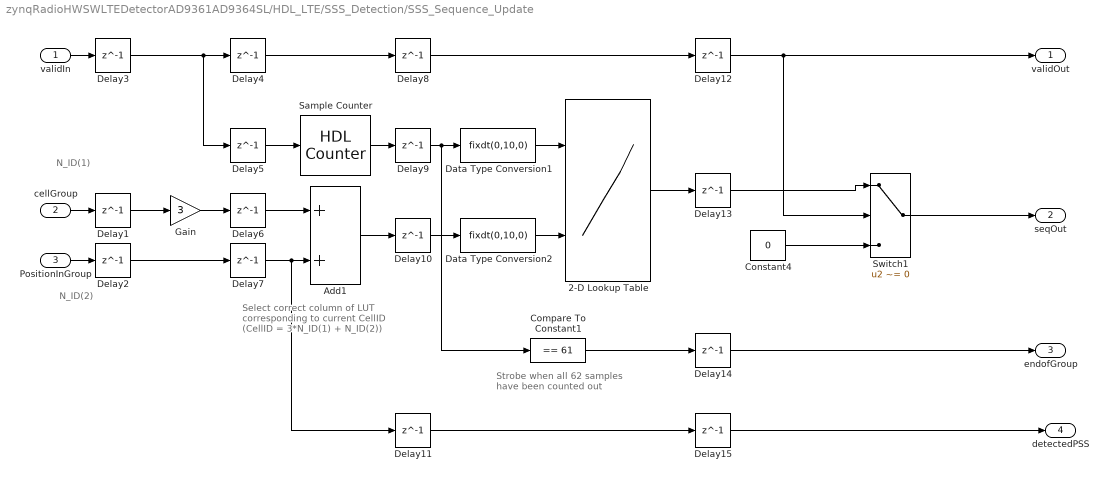
== system zynqRadioHWSWLTEDetectorAD9361AD9364SL/HDL_LTE/SSS_Detection/SSS_Sequence_Update ==
  note: N_ID(2)
  note: Select correct column of LUT
      | corresponding to current CellID
      | (CellID = 3*N_ID(1) + N_ID(2))
  note: N_ID(1)
  note: Strobe when all 62 samples
      | have been counted out
  validIn : Inport
  cellGroup : Inport  Port=2
  PositionInGroup : Inport  Port=3
  2-D Lookup Table : Lookup_n-D  BreakpointsForDimension1=[0:size(simParams.possibleSSS,1)-1]  BreakpointsForDimension2=[0:size(simParams.possibleSSS,2)-1]  IndexSearchMethod=Evenly spaced points  Table=real(simParams.possibleSSS)  TableDataTypeStr=fixdt(1,2,0)  InterpMethod=Flat  DiagnosticForOutOfRangeInput=Error  InternalRulePriority=Speed  OutDataTypeStr=fixdt(1,2,0)  RndMeth=Simplest  InputSameDT=on
  Add1 : Sum  OutDataTypeStr=Inherit: Same as first input
  Compare To Constant1 : simulink/Logic and Bit Operations/Compare To Constant  relop===  const=61  OutDataTypeStr=boolean
  Constant4 : Constant  Value=0  OutDataTypeStr=fixdt(1,2,0)  SampleTime=simParams.TsRx
  Data Type Conversion1 : DataTypeConversion  OutDataTypeStr=fixdt(0,10,0)
  Data Type Conversion2 : DataTypeConversion  OutDataTypeStr=fixdt(0,10,0)
  Delay{1..15} (15 alike) : Delay  DelayLength=1  InitialCondition=0
  Gain : Gain  Gain=3  OutDataTypeStr=fixdt(0,10,0)
  Sample Counter : hdlsllib/HDL Operations/HDL Counter  CountType=Count limited  CountInit=0  CountStep=1  CountMax=61  CountFromType=Initial value  CountFrom=0  CountResetPort=off  CountLoadPort=off  CountEnbPort=on  CountDirPort=off  CountDataType=Unsigned  CountWordLen=ceil(log2(61))  CountFracLen=0  CountSampTime=1
  Switch1 : Switch  Criteria=u2 ~= 0
  validOut : Outport  InitialOutput=0
  seqOut : Outport  Port=2  InitialOutput=0
  endofGroup : Outport  Port=3  InitialOutput=0
  detectedPSS : Outport  Port=4  InitialOutput=0
  wires:
  Constant4/1 -> Switch1/3
  Data Type Conversion1/1 -> 2-D Lookup Table/1
  Data Type Conversion2/1 -> 2-D Lookup Table/2
  2-D Lookup Table/1 -> Delay13/1
  Compare To Constant1/1 -> Delay14/1
  cellGroup/1 -> Delay1/1
  Gain/1 -> Delay6/1
  validIn/1 -> Delay3/1
  Sample Counter/1 -> Delay9/1
  Add1/1 -> Delay10/1
  PositionInGroup/1 -> Delay2/1
  Delay3/1 -> Delay4/1, Delay5/1
  Delay1/1 -> Gain/1
  Delay2/1 -> Delay7/1
  Delay4/1 -> Delay8/1
  Delay5/1 -> Sample Counter/1
  Delay6/1 -> Add1/1
  Delay7/1 -> Delay11/1, Add1/2
  Delay8/1 -> Delay12/1
  Delay9/1 -> Data Type Conversion1/1, Compare To Constant1/1
  Delay10/1 -> Data Type Conversion2/1
  Delay11/1 -> Delay15/1
  Delay12/1 -> validOut/1, Switch1/2
  Delay13/1 -> Switch1/1
  Switch1/1 -> seqOut/1
  Delay14/1 -> endofGroup/1
  Delay15/1 -> detectedPSS/1

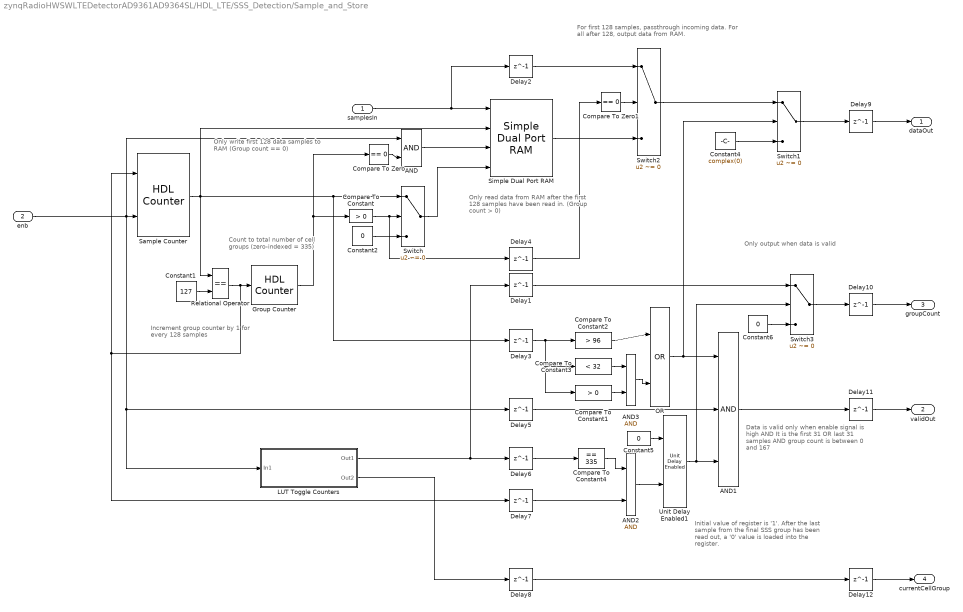
== system zynqRadioHWSWLTEDetectorAD9361AD9364SL/HDL_LTE/SSS_Detection/Sample_and_Store ==
  note: Count to total number of
      | cell groups
      | (zero-indexed = 335)
  note: For first 128 samples, passthrough incoming data.
      | For all after 128, output data from RAM.
  note: Data is valid only when enable
      | signal is high AND It is the first
      | 31 OR last 31 samples AND
      | group count is between 0 and 167
  note: Only read data from RAM after the
      | first 128 samples have been read in.
      | (Group count > 0)
  note: Only write first 128 data samples
      | to RAM (Group count == 0)
  note: Increment group counter by 1
      | for every 128 samples
  note: Initial value of register is '1'.
      | After the last sample from the
      | final SSS group has been read out,
      | a '0' value is loaded into the register.
  note: Only output when data is valid
  samplesIn : Inport
  enb : Inport  Port=2
  AND : Logic  IconShape=distinctive  AllPortsSameDT=off  OutDataTypeStr=boolean
  AND1 : Logic  Inputs=3  IconShape=distinctive  AllPortsSameDT=off  OutDataTypeStr=boolean
  AND2 : Logic  IconShape=distinctive  AllPortsSameDT=off  OutDataTypeStr=boolean
  AND3 : Logic  IconShape=distinctive  AllPortsSameDT=off  OutDataTypeStr=boolean
  Compare To Constant : simulink/Logic and Bit Operations/Compare To Constant  relop=>  const=0  OutDataTypeStr=boolean
  Compare To Constant1 : simulink/Logic and Bit Operations/Compare To Constant  relop=>  const=0  OutDataTypeStr=boolean
  Compare To Constant2 : simulink/Logic and Bit Operations/Compare To Constant  relop=>  const=96  OutDataTypeStr=boolean
  Compare To Constant3 : simulink/Logic and Bit Operations/Compare To Constant  relop=<  const=32  OutDataTypeStr=boolean
  Compare To Constant4 : simulink/Logic and Bit Operations/Compare To Constant  relop===  const=335  OutDataTypeStr=boolean
  Compare To Zero : simulink/Logic and Bit Operations/Compare To Zero  relop===  OutDataTypeStr=boolean
  Compare To Zero1 : simulink/Logic and Bit Operations/Compare To Zero  relop===  OutDataTypeStr=boolean
  Constant1 : Constant  Value=127  OutDataTypeStr=fixdt(0,8,0)  SampleTime=simParams.TsRx
  Constant2 : Constant  Value=0  OutDataTypeStr=fixdt(0,7,0)  SampleTime=simParams.TsRx
  Constant4 : Constant  Value=complex(0)  OutDataTypeStr=Inherit: Inherit via back propagation  SampleTime=simParams.TsRx
  Constant5 : Constant  Value=0  OutDataTypeStr=boolean  SampleTime=simParams.TsRx
  Constant6 : Constant  Value=0  OutDataTypeStr=fixdt(0,9,0)  SampleTime=simParams.TsRx
  Delay{1..12} (12 alike) : Delay  DelayLength=1  InitialCondition=0
  Group Counter : hdlsllib/HDL Operations/HDL Counter  CountType=Count limited  CountInit=0  CountStep=1  CountMax=335  CountFromType=Initial value  CountFrom=0  CountResetPort=off  CountLoadPort=off  CountEnbPort=on  CountDirPort=off  CountDataType=Unsigned  CountWordLen=ceil(log2(335))  CountFracLen=0  CountSampTime=1
  LUT Toggle Counters : Subsystem
  OR : Logic  Operator=OR  IconShape=distinctive  AllPortsSameDT=off  OutDataTypeStr=boolean
  Relational Operator : RelationalOperator  Operator===  OutDataTypeStr=boolean
  Sample Counter : hdlsllib/HDL Operations/HDL Counter  CountType=Count limited  CountInit=0  CountStep=1  CountMax=127  CountFromType=Initial value  CountFrom=0  CountResetPort=on  CountLoadPort=off  CountEnbPort=on  CountDirPort=off  CountDataType=Unsigned  CountWordLen=log2(128)  CountFracLen=0  CountSampTime=1
  Simple Dual Port RAM : hdlsllib/HDL Operations/Simple Dual Port RAM  ram_size=7
  Switch : Switch  Criteria=u2 ~= 0
  Switch1 : Switch  Criteria=u2 ~= 0  InputSameDT=on
  Switch2 : Switch  Criteria=u2 ~= 0
  Switch3 : Switch  Criteria=u2 ~= 0
  Unit Delay Enabled1 : simulink/Additional Math & Discrete/Additional Discrete/Unit Delay Enabled  vinit=1  tsamp=-1
  dataOut : Outport
  validOut : Outport  Port=2
  groupCount : Outport  Port=3
  currentCellGroup : Outport  Port=4
  wires:
  Compare To Constant1/1 -> AND3/2
  Compare To Constant3/1 -> AND3/1
  AND3/1 -> OR/2
  Constant6/1 -> Switch3/3
  Delay7/1 -> AND2/2
  Unit Delay Enabled1/1 -> AND1/3, Switch3/2
  AND2/1 -> Unit Delay Enabled1/2
  Constant5/1 -> Unit Delay Enabled1/1
  samplesIn/1 -> Simple Dual Port RAM/1, Delay2/1
  Delay5/1 -> AND1/2
  Delay4/1 -> Compare To Zero1/1
  Delay3/1 -> Compare To Constant3/1, Compare To Constant1/1, Compare To Constant2/1
  Delay2/1 -> Switch2/1
  Switch2/1 -> Switch1/1
  Simple Dual Port RAM/1 -> Switch2/3
  Compare To Zero1/1 -> Switch2/2
  Constant4/1 -> Switch1/3
  OR/1 -> AND1/1, Switch1/2
  Compare To Constant2/1 -> OR/1
  Constant2/1 -> Switch/3
  Switch/1 -> Simple Dual Port RAM/4
  Compare To Zero/1 -> AND/2
  Compare To Constant/1 -> Switch/2, Delay4/1
  AND/1 -> Simple Dual Port RAM/3
  Constant1/1 -> Relational Operator/2
  enb/1 -> AND/1, Delay5/1, LUT Toggle Counters/1(In1), Sample Counter/2
  Group Counter/1 -> Compare To Constant/1, Compare To Zero/1
  Sample Counter/1 -> Switch/1, Delay3/1, Relational Operator/1, Simple Dual Port RAM/2
  Delay1/1 -> Switch3/1
  LUT Toggle Counters/1(Out1) -> Delay6/1, Delay1/1
  Delay6/1 -> Compare To Constant4/1
  Compare To Constant4/1 -> AND2/1
  Relational Operator/1 -> Group Counter/1, Delay7/1, Sample Counter/1
  Switch1/1 -> Delay9/1
  Switch3/1 -> Delay10/1
  AND1/1 -> Delay11/1
  LUT Toggle Counters/2(Out2) -> Delay8/1
  Delay8/1 -> Delay12/1
  Delay9/1 -> dataOut/1
  Delay10/1 -> groupCount/1
  Delay11/1 -> validOut/1
  Delay12/1 -> currentCellGroup/1

== system zynqRadioHWSWLTEDetectorAD9361AD9364SL/HDL_LTE/Frequency_Estimation/Cyclic_Prefix_Correlator/Moving_Average ==
  note: Use a comb filter followed by an integrator
      | to implement an efficient 9-tab moving average.
  dataIn : Inport
  Add : Sum  Inputs=-+  AccumDataTypeStr=fixdt(1,27,23)
  Add1 : Sum  AccumDataTypeStr=fixdt(1,27,23)
  Delay1 : Delay  DelayLength=8  InitialCondition=0
  Delay10 : Delay  DelayLength=1  InitialCondition=0  UseCircularBuffer=on
  Delay2 : Delay  DelayLength=1  InitialCondition=0  UseCircularBuffer=on
  Delay3 : Delay  DelayLength=1  InitialCondition=0  UseCircularBuffer=on
  Gain : Gain  Gain=1/8  OutDataTypeStr=fixdt(1,24,23)
  dataOut : Outport
  wires:
  Add/1 -> Delay10/1
  dataIn/1 -> Add/2, Delay1/1
  Delay1/1 -> Add/1
  Add1/1 -> Delay2/1
  Delay10/1 -> Add1/2
  Delay2/1 -> Gain/1, Add1/1
  Gain/1 -> Delay3/1
  Delay3/1 -> dataOut/1

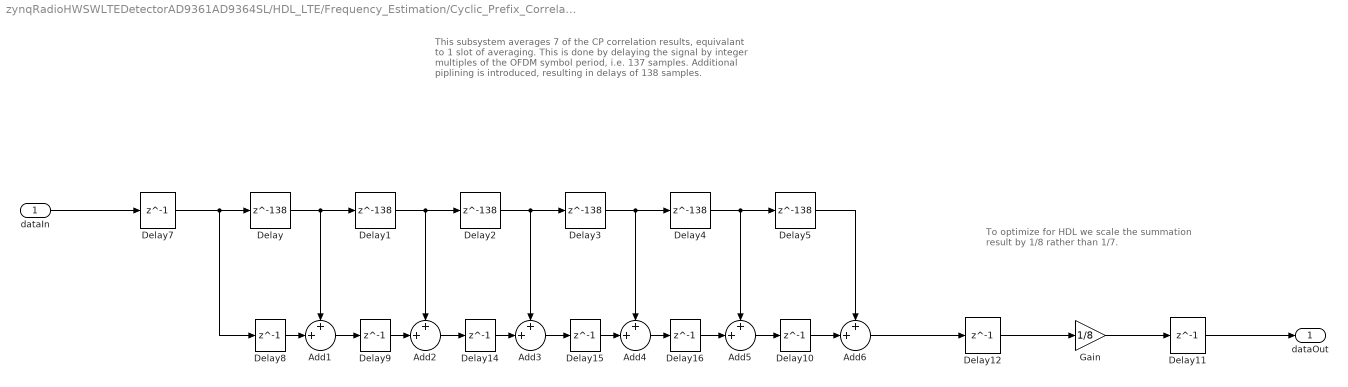
== system zynqRadioHWSWLTEDetectorAD9361AD9364SL/HDL_LTE/Frequency_Estimation/Cyclic_Prefix_Correlator/Slot_Average ==
  note: This subsystem averages 7 of the CP correlation results, equivalant to 1 slot of averaging. This is done by delaying the signal by integer multiples of the OFDM symbol period, i.e. 137 samples.
      |
      | Additional piplining is introduced, resulting in delays of 138 samples.
  note: To optimize for HDL we scale the summation result by 1/8 rather than 1/7.
  dataIn : Inport
  Add1 : Sum  Inputs=++|  AccumDataTypeStr=fixdt(1,28,23)
  Add2 : Sum  Inputs=++|  AccumDataTypeStr=fixdt(1,29,23)
  Add3 : Sum  Inputs=++|  OutDataTypeStr=fixdt(1,29,23)
  Add4 : Sum  Inputs=++|  AccumDataTypeStr=fixdt(1,29,23)
  Add5 : Sum  Inputs=++|  AccumDataTypeStr=fixdt(1,30,23)
  Add6 : Sum  Inputs=++|  AccumDataTypeStr=fixdt(1,30,23)
  Delay{,1..5} (6 alike) : Delay  DelayLength=138  InitialCondition=0
  Delay{7..12,14..16} (9 alike) : Delay  DelayLength=1  InitialCondition=0  UseCircularBuffer=on
  Gain : Gain  Gain=1/8  OutDataTypeStr=fixdt(1,24,23)
  dataOut : Outport
  wires:
  Delay4/1 -> Delay5/1, Add5/1
  Delay/1 -> Delay1/1, Add1/1
  Add1/1 -> Delay9/1
  Delay1/1 -> Delay2/1, Add2/1
  Delay3/1 -> Delay4/1, Add4/1
  Delay2/1 -> Delay3/1, Add3/1
  dataIn/1 -> Delay7/1
  Add2/1 -> Delay14/1
  Add3/1 -> Delay15/1
  Add4/1 -> Delay16/1
  Add5/1 -> Delay10/1
  Delay5/1 -> Add6/1
  Add6/1 -> Delay12/1
  Delay7/1 -> Delay8/1, Delay/1
  Delay8/1 -> Add1/2
  Delay9/1 -> Add2/2
  Delay14/1 -> Add3/2
  Delay15/1 -> Add4/2
  Delay16/1 -> Add5/2
  Delay10/1 -> Add6/2
  Delay12/1 -> Gain/1
  Gain/1 -> Delay11/1
  Delay11/1 -> dataOut/1

== system zynqRadioHWSWLTEDetectorAD9361AD9364SL/HDL_LTE/PSS_Detection/Cross_Correlation/Averaging_Filter ==
  datIn : Inport
  Add : Sum  Inputs=-+  AccumDataTypeStr=fixdt(1,32,23)  OutDataTypeStr=Inherit: Same as accumulator
  Add1 : Sum  AccumDataTypeStr=fixdt(1,32,23)  OutDataTypeStr=Inherit: Same as accumulator
  Delay1 : Delay  DelayLength=128  InitialCondition=0
  Delay2 : Delay  DelayLength=1  InitialCondition=0  UseCircularBuffer=on
  Delay3 : Delay  DelayLength=1  InitialCondition=0  UseCircularBuffer=on
  Gain : Gain  Gain=2^-7  OutDataTypeStr=fixdt(1,25,23)
  thresholdOut : Outport
  wires:
  Delay3/1 -> Add1/2
  Add1/1 -> Delay2/1
  Add/1 -> Delay3/1
  Delay2/1 -> Gain/1, Add1/1
  Delay1/1 -> Add/1
  datIn/1 -> Add/2, Delay1/1
  Gain/1 -> thresholdOut/1

== system zynqRadioHWSWLTEDetectorAD9361AD9364SL/HDL_LTE/PSS_Detection/Cross_Correlation/Magnitude_Squared ==
  dataIn : Inport
  Add : Sum  OutDataTypeStr=Inherit: Same as accumulator
  Complex to Real-Imag : ComplexToRealImag
  Data Type Conversion : DataTypeConversion  OutDataTypeStr=fixdt(1,25,23)  RndMeth=Round
  Delay1 : Delay  InitialCondition=0
  Delay2 : Delay  InitialCondition=0
  Delay3 : Delay  DelayLength=1  InitialCondition=0
  Delay4 : Delay  DelayLength=1  InitialCondition=0
  Delay5 : Delay  DelayLength=1  InitialCondition=0
  Product1 : Product
  Product4 : Product
  Magnitude^2 : Outport
  wires:
  Delay4/1 -> Data Type Conversion/1
  Delay2/1 -> Add/1
  Delay1/1 -> Add/2
  Delay3/1 -> Complex to Real-Imag/1
  dataIn/1 -> Delay3/1
  Product4/1 -> Delay2/1
  Complex to Real-Imag/2 -> Product1/1, Product1/2
  Complex to Real-Imag/1 -> Product4/1, Product4/2
  Add/1 -> Delay4/1
  Product1/1 -> Delay1/1
  Delay5/1 -> Magnitude^2/1
  Data Type Conversion/1 -> Delay5/1
